simulink model "mcb_ipmsm_pos_est_f28379d"  (R2023b)
settings: Solver=FixedStepDiscrete  StartTime=0.0  StopTime=1  RelTol=1e-3  EnableMultiTasking=on
InitFcn:
  | mcb_ipmsm_pos_est_f28379d_data;
  | init_ang = eval(get_param([bdroot '/Inverter and Motor/Simulation/Init angle'],'Value'))/pmsm.p;
values from neighbouring files (symbols this model uses):
  dataType = 'single'    [mcb_ipmsm_pos_est_f28379d_data.m]
  inverter = mcb_updateInverterParameters(pmsm,inverter,target)    [mcb_ipmsm_pos_est_f28379d_data.m]
  pmsm = mcb_SetPMSMMotorParameters('Teknic2310P')    [mcb_ipmsm_pos_est_f28379d_data.m]
  PWM_frequency = 20e3    (= 20000)    [mcb_ipmsm_pos_est_f28379d_data.m]
  target = mcb_SetProcessorDetails('F28379D',PWM_frequency)    [mcb_ipmsm_pos_est_f28379d_data.m]
  Ts = T_pwm    (= 5e-05)    [mcb_ipmsm_pos_est_f28379d_data.m]
  Ts_motor_simscape = T_pwm/2000    (= 2.5e-08)    [mcb_ipmsm_pos_est_f28379d_data.m]
  Ts_simulink = T_pwm/2    (= 2.5e-05)    [mcb_ipmsm_pos_est_f28379d_data.m]
undefined symbols (not defined in the file or in its folder): Down, GPTRIP1SEL, GPTRIP2SEL, PU_System, TZ1, TZ2, Up
libraries: nesl_utility x12, c2802xlib x7, fl_lib x7, c280xlib x5, ee_lib x5, c2837xDlib x4, simulink x3, svdschedulerlib x1, mcbcontrolslib x1, mcbsensorlessestimatorlib x1, svdutilitieslib x1, mcbpositiondecoderlib x1
(part 1 of 2)
settings Model: ExtModeTrigDuration=8  Creator=The MathWorks, Inc.  LastModifiedBy=The MathWorks, Inc.
settings SolverCC: AlgebraicLoopSolver=TrustRegion  MaxZcPerStep=1
settings DataIOCC: ReturnWorkspaceOutputs=off
settings OptimizationCC: DefaultParameterBehavior=Inlined  DefaultUnderspecifiedDataType=single  OptimizeBlockIOStorage=off  ReuseModelBlockBuffer=off  EnhancedBackFolding=on  InitFltsAndDblsToZero=on  NoFixptDivByZeroProtection=on  EfficientFloat2IntCast=on  EfficientMapNaN2IntZero=off  MaxStackSize=1024  OptimizeBlockOrder=speed  DifferentSizesBufferReuse=on  DenormalBehavior=FlushToZero  EfficientTunableParamExpr=on
settings DebuggingCC: ReadBeforeWriteMsg=DisableAll  WriteAfterWriteMsg=DisableAll  WriteAfterReadMsg=DisableAll  InheritedTsInSrcMsg=none  MultiTaskDSMMsg=none  ParameterPrecisionLossMsg=none  ParameterTunabilityLossMsg=error  UnconnectedInputMsg=warning  UnconnectedOutputMsg=warning  UnconnectedLineMsg=warning
settings HardwareCC: ProdBitPerChar=16  ProdBitPerInt=16  ProdBitPerPointer=32  ProdBitPerSizeT=32  ProdBitPerPtrDiffT=32  ProdLargestAtomicInteger=Integer  ProdLargestAtomicFloat=None  ProdWordSize=16  ProdLongLongMode=on  ProdHWDeviceType=Texas Instruments->C2000
settings ModelReferenceCC: EnableRefExpFcnMdlSchedulingChecks=on
settings SFSimCC: MATLABDynamicMemAlloc=off
settings RTWCC: Description=Embedded Coder  SystemTargetFile=ert.tlc  HardwareBoard=TI Delfino F28379D LaunchPad  TemplateMakefile=ert_default_tmf  GenerateReport=on  Toolchain=Texas Instruments Code Composer Studio (C2000)  DLArmComputeVersion=19.05
settings CodeAppCC: IgnoreCustomStorageClasses=off  StateflowObjectComments=on
settings ERTTargetCC: CodeReplacementLibrary=TI C28x  ExtModeStaticAllocSize=10000  ConvertIfToSwitch=off  SuppressUnreachableDefaultCases=off  MemSecPackage=tic2000demospkg

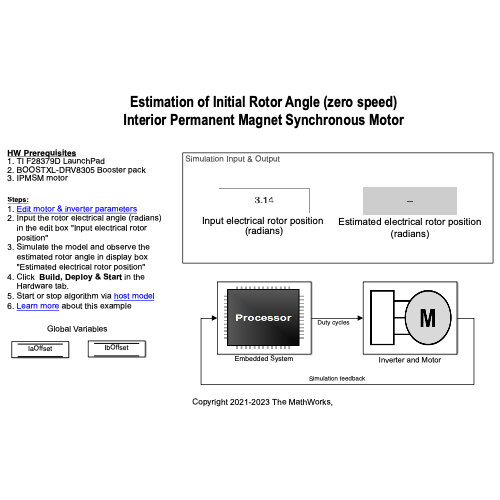
[thumbnail: Simulink's stored preview of the top-level diagram]
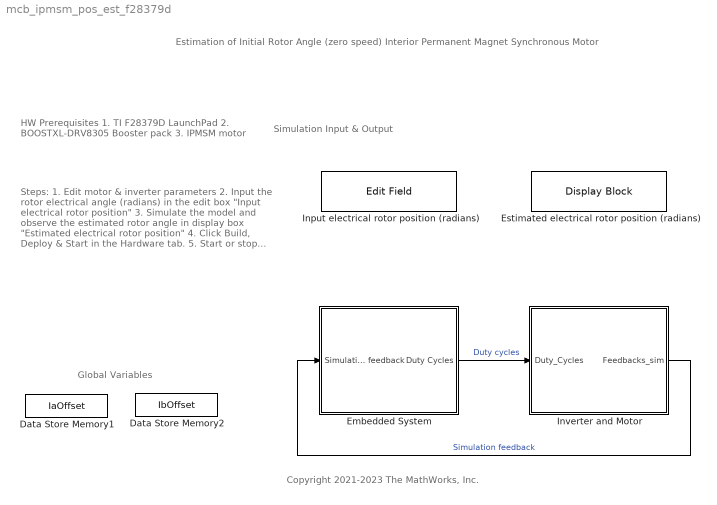
== system mcb_ipmsm_pos_est_f28379d ==
  note: Estimation of Initial Rotor Angle (zero speed)
      | Interior Permanent Magnet Synchronous Motor
  note: Simulation Input & Output
  note: Steps:
      | 1. Edit motor & inverter parameters
      | 2. Input the rotor electrical angle (radians)
      | in the edit box "Input electrical rotor
      | position"
      | 3. Simulate the model and observe the
      | estimated rotor angle in display box
      | "Estimated electrical rotor position"
      | 4. Click Build, Deploy & Start in the
      | Hardware tab.
      | 5. Start or stop algorithm via host model
      | 6. Learn more about this example
  note: HW Prerequisites
      | 1. TI F28379D LaunchPad
      | 2. BOOSTXL-DRV8305 Booster pack
      | 3. IPMSM motor
  note: Global Variables
  note: Copyright 2021-2023 The MathWorks, Inc.
  Data Store Memory1 : DataStoreMemory  DataStoreName=IaOffset  InitialValue=inverter.CtSensAOffset  ShowAdditionalParam=off
  Data Store Memory2 : DataStoreMemory  DataStoreName=IbOffset  InitialValue=inverter.CtSensBOffset  ShowAdditionalParam=off
  Embedded System : Subsystem
      mask Display: image('mcb_pmsmfoc_processor.png'); % Use "Edit Image" on toolstrip to change.
  Estimated electrical rotor position (radians) : DisplayBlock  LabelPosition=Hide  Transparency=1  FormatString=%5d
  Input electrical rotor position (radians) : EditField  LabelPosition=Hide  ShowInitialText=on  Alignment=Center
  Inverter and Motor : Subsystem
      mask Display: image('mcb_pmsmfoc_motor.png'); % Use "Edit Image" on toolstrip to change.
  wires:
  Inverter and Motor/1(Feedbacks_sim) -> Embedded System/1(Simulation feedback)  "Simulation feedback"
  Embedded System/1(Duty Cycles) -> Inverter and Motor/1(Duty_Cycles)  "Duty cycles"

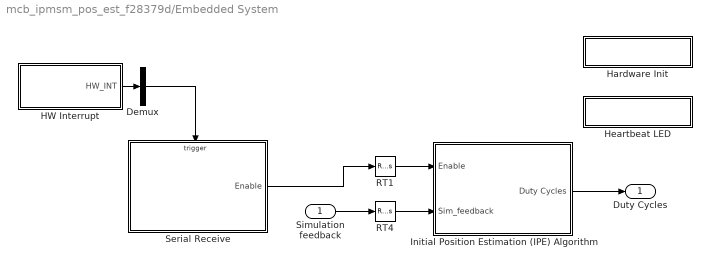
== system mcb_ipmsm_pos_est_f28379d/Embedded System ==
  Simulation feedback : Inport
  Demux : Demux  Outputs=1
  HW Interrupt : Subsystem  Variant=on  VariantControlMode=sim codegen switching
  Hardware Init : Subsystem  TreatAsAtomicUnit=on
  Heartbeat LED : Subsystem  TreatAsAtomicUnit=on
  Initial Position Estimation (IPE) Algorithm : Subsystem
      settings: RTWSystemCode=Nonreusable function
  RT1 : RateTransition  Deterministic=off  OutPortSampleTime=Ts
  RT4 : RateTransition  Deterministic=off  OutPortSampleTime=Ts
  Serial Receive : Subsystem  SystemSampleTime=1e-3
  Duty Cycles : Outport
  wires:
  HW Interrupt/1(HW_INT) -> Demux/1
  RT4/1 -> Initial Position Estimation (IPE) Algorithm/2(Sim_feedback)
  Initial Position Estimation (IPE) Algorithm/1(Duty Cycles) -> Duty Cycles/1
  Simulation feedback/1 -> RT4/1
  Demux/1 -> Serial Receive/Trigger
  Serial Receive/1(Enable) -> RT1/1
  RT1/1 -> Initial Position Estimation (IPE) Algorithm/1(Enable)

== system mcb_ipmsm_pos_est_f28379d/Inverter and Motor ==
  Duty_Cycles : Inport
  Codegeneration : Subsystem
  Simulation : Subsystem
  Variant Sink : VariantSink  VariantControlMode=sim codegen switching
  Variant Source : VariantSource  VariantControlMode=sim codegen switching
  Feedbacks_sim : Outport  VectorParamsAs1DForOutWhenUnconnected=off
  wires:
  Duty_Cycles/1 -> Variant Sink/1
  Variant Source/1 -> Feedbacks_sim/1
  Variant Sink/2 -> Simulation/1(Duty_Cycles)
  Simulation/1(Feedbacks) -> Variant Source/2
  Variant Sink/1 -> Codegeneration/1(Duty_Cycles)
  Codegeneration/1(Feedbacks) -> Variant Source/1

== system mcb_ipmsm_pos_est_f28379d/Embedded System/HW Interrupt ==
  Code generation : Subsystem  VariantControl=(codegen)
  Simulation : Subsystem  VariantControl=(sim)
  HW_INT : Outport  OutputFunctionCall=on

== system mcb_ipmsm_pos_est_f28379d/Embedded System/Hardware Init ==
  6PWM_Mode : Constant  Priority=1000  Value=0x3A16  OutDataTypeStr=uint16  SampleTime=-1
  ADC_Gain_Setting : Constant  Priority=1000  Value=inverter.SPI_Gain_Setting  OutDataTypeStr=uint16  SampleTime=-1
  Event Listener : EventListener  DisableCoverage=on  EventName=reset
  Mux : Mux  Inputs=2
  Variant Subsystem : Subsystem  Variant=on  VariantControlMode=sim codegen switching
  wires:
  6PWM_Mode/1 -> Mux/1
  ADC_Gain_Setting/1 -> Mux/2
  Mux/1 -> Variant Subsystem/1(In1)

== system mcb_ipmsm_pos_est_f28379d/Embedded System/Heartbeat LED ==
  note: Heartbeat LED 1HZ
  Heartbeat LED : Subsystem  Variant=on  VariantControlMode=sim codegen switching
  RED_LED : Constant  OutDataTypeStr=uint16  SampleTime=0.5
  wires:
  RED_LED/1 -> Heartbeat LED/1(In1)

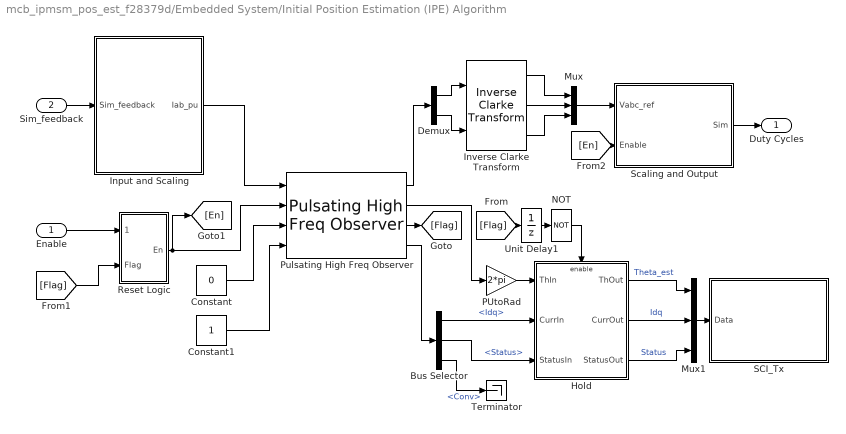
== system mcb_ipmsm_pos_est_f28379d/Embedded System/Initial Position Estimation (IPE) Algorithm ==
  Enable : Inport
  Sim_feedback : Inport  Port=2
  Bus Selector : BusSelector  OutputSignals=Idq,Status,Conv
  Constant : Constant  Value=0  OutDataTypeStr=dataType
  Constant1 : Constant  OutDataTypeStr=boolean
  Demux : Demux  Outputs=2
  Hold : Subsystem
  Input and Scaling : Subsystem
  Inverse Clarke Transform : mcbcontrolslib/Inverse Clarke Transform  PhaseInput=Two inputs  EnPowerInv=off
  Mux : Mux  Inputs=3
  Mux1 : Mux  Inputs=3
  NOT : Logic  Operator=NOT  IconShape=distinctive  AllPortsSameDT=off  OutDataTypeStr=boolean
  PUtoRad : Gain  Gain=2*pi  OutDataTypeStr=Inherit: Same as input
  Pulsating High Freq Observer : mcbsensorlessestimatorlib/Pulsating High Freq Observer  BlkSampleTime=Ts  InputUnit=Per-unit  dataType=dataType  AutoDefaultPHF=off  AutoDefaultDP=off  StatorResistance=pmsm.Rs  StatorDaxisInductance=pmsm.Ld  StatorQaxisInductance=pmsm.Lq  BaseVoltage=PU_System.V_base  BaseCurrent=PU_System.I_base  Voltphf=0.5  Frqphf=2000  Cfrqphf=131.9037  SelectForTuning=Controller gains  Kp=1954.6647  Ki=7392.5303  Tsettling=0.66794  DampingRatio=0.99  Tophf=0.0066794  Tcphf=0.66794  Idlephf=0.0066794  Threshold=4e-4  Voltdp=0.5  Tdp=0.00066955  Idledp=50e-3  PHF_OpenLoop=134  PHF_Period=10  PHF_Delay=134  PHF_OL_Total=804  PHF_CloseLoop=13359  PHF_Total=14297  DP_On=14  DP_Delay=1000  DP_Total=0  IPE_Total=16325  DefaultCal=0
      settings: RTWMemSecFuncExecute=code_ramfuncs
  Reset Logic : Subsystem
  SCI_Tx : Subsystem  Variant=on  VariantControlMode=sim codegen switching
  Scaling and Output : Subsystem
  Terminator : Terminator
  Unit Delay1 : UnitDelay  SampleTime=-1  HasFrameUpgradeWarning=on
  Duty Cycles : Outport  InitialOutput=0  VectorParamsAs1DForOutWhenUnconnected=off
  wires:
  Mux1/1 -> SCI_Tx/1(Data)
  Sim_feedback/1 -> Input and Scaling/1(Sim_feedback)
  Scaling and Output/1(Sim) -> Duty Cycles/1
  Inverse Clarke Transform/1 -> Mux/1
  Inverse Clarke Transform/2 -> Mux/2
  Inverse Clarke Transform/3 -> Mux/3
  Mux/1 -> Scaling and Output/1(Vabc_ref)
  Demux/1 -> Inverse Clarke Transform/1
  Demux/2 -> Inverse Clarke Transform/2
  Pulsating High Freq Observer/1 -> Demux/1
  [En] -> Scaling and Output/2(Enable)
  Input and Scaling/1(Iab_pu) -> Pulsating High Freq Observer/1
  Pulsating High Freq Observer/2 -> PUtoRad/1
  Hold/1(ThOut) -> Mux1/1  "Theta_est"
  NOT/1 -> Hold/Enable
  Constant/1 -> Pulsating High Freq Observer/3
  Constant1/1 -> Pulsating High Freq Observer/4
  Pulsating High Freq Observer/4 -> Bus Selector/1
  Pulsating High Freq Observer/3 -> [Flag]
  Enable/1 -> Reset Logic/1(Enable)
  [Flag] -> Reset Logic/2(Flag)
  Reset Logic/1(En) -> Pulsating High Freq Observer/2, [En]
  Bus Selector/1 -> Hold/2(CurrIn)  "<Idq>"
  Bus Selector/2 -> Hold/3(StatusIn)  "<Status>"
  Hold/3(StatusOut) -> Mux1/3  "Status"
  [Flag] -> Unit Delay1/1
  Unit Delay1/1 -> NOT/1
  Hold/2(CurrOut) -> Mux1/2  "Idq"
  Bus Selector/3 -> Terminator/1  "<Conv>"
  PUtoRad/1 -> Hold/1(ThIn)

== system mcb_ipmsm_pos_est_f28379d/Embedded System/Serial Receive ==
  SCI_Rx_INT : TriggerPort  TriggerType=function-call  VariantControl=Variant
  Data Type Conversion1 : DataTypeConversion  OutDataTypeStr=boolean  RndMeth=Simplest  SaturateOnIntegerOverflow=off
  Data_Conditioning_Rx : Subsystem  Variant=on
  SCi_Rx : Subsystem  Variant=on  VariantControlMode=sim codegen switching
  Enable : Outport
  wires:
  SCi_Rx/1(Data) -> Data_Conditioning_Rx/1(In1)
  Data_Conditioning_Rx/1(Out3) -> Data Type Conversion1/1
  Data Type Conversion1/1 -> Enable/1

== system mcb_ipmsm_pos_est_f28379d/Inverter and Motor/Codegeneration ==
  Duty_Cycles : Inport
  Ground : Ground
  Terminator : Terminator
  Feedbacks : Outport  VectorParamsAs1DForOutWhenUnconnected=off
  wires:
  Duty_Cycles/1 -> Terminator/1
  Ground/1 -> Feedbacks/1

== system mcb_ipmsm_pos_est_f28379d/Inverter and Motor/Simulation ==
  note: "Initi angle" constant is connected with user input " Input electrical rotor
      | position " to define initial rotor position for PMSM motor block
  Duty_Cycles : Inport
  Constant : Constant  Value=0  OutDataTypeStr=dataType
  Data Type Conversion : DataTypeConversion  OutDataTypeStr=single  RndMeth=Simplest  SaturateOnIntegerOverflow=off
  Init angle : Constant  Value=3.14  OutDataTypeStr=dataType
  Inveter and Motor : Subsystem  VariantControl=(get_param([bdroot '/MotorWindingType'], 'Value') == '1')
  RT1 : RateTransition  Deterministic=off  OutPortSampleTime=Ts_simulink
  Sensor_Measurements : Subsystem
  Terminator2 : Terminator
  Feedbacks : Outport  VectorParamsAs1DForOutWhenUnconnected=off
  wires:
  Sensor_Measurements/1(Sim_fb) -> Feedbacks/1
  RT1/1 -> Sensor_Measurements/1(PhaseCurr)
  Duty_Cycles/1 -> Data Type Conversion/1
  Constant/1 -> Inveter and Motor/2(Load)
  Inveter and Motor/1(Iabc) -> RT1/1
  Init angle/1 -> Terminator2/1
  Data Type Conversion/1 -> Inveter and Motor/1(Vabc_In_PU)

== system mcb_ipmsm_pos_est_f28379d/Embedded System/HW Interrupt/Code generation ==
  HWI_SCIA_RX_INT : svdschedulerlib/Hardware Interrupt v2  ISRGroup=ADC - Analog to Digital Converter  ISRName=ADCA1_INT  ISRNumber=32  NumEventsToServe=1  EventsList={'on','EOC event','1';'off','Overflow event','2';'off','Custom event','3'}  SelectedEvents={'event1'}  TaskPriority=50  DisablePreemption=on  ClearInterruptFlagsAtEndOfEvent=on  InterruptDefinitionFile=$(TARGET_ROOT)/registry/interrupts/F2837xS_interrupts.xml  HardwareBoard=F2837x  EnableSimPort=off
      settings: LibrarySourceBlock=c2000lib/Scheduling/Hardware Interrupt
  HW_INT : Outport
  wires:
  HWI_SCIA_RX_INT/1 -> HW_INT/1

== system mcb_ipmsm_pos_est_f28379d/Embedded System/HW Interrupt/Simulation ==
  SCI_Rx_INT : simulink/Ports & Subsystems/Function-Call Generator  sample_time=0.1  numberOfIterations=1  DisallowWideOutput=off
  HW_INT : Outport
  wires:
  SCI_Rx_INT/1 -> HW_INT/1

== system mcb_ipmsm_pos_est_f28379d/Embedded System/Hardware Init/Variant Subsystem ==
  In1 : Inport
  Code Generation : Subsystem  VariantControl=(codegen)
  Simulation : Subsystem  VariantControl=(sim)

== system mcb_ipmsm_pos_est_f28379d/Embedded System/Heartbeat LED/Heartbeat LED ==
  In1 : Inport
  Code generation : Subsystem  VariantControl=(codegen)
  Simulation : Subsystem  VariantControl=(sim)

== system mcb_ipmsm_pos_est_f28379d/Embedded System/Initial Position Estimation (IPE) Algorithm/Hold ==
  ThIn : Inport
  CurrIn : Inport  Port=2
  StatusIn : Inport  Port=3
  Enable : EnablePort
  ThOut : Outport
  CurrOut : Outport  Port=2
  StatusOut : Outport  Port=3
  wires:
  ThIn/1 -> ThOut/1
  CurrIn/1 -> CurrOut/1
  StatusIn/1 -> StatusOut/1

== system mcb_ipmsm_pos_est_f28379d/Embedded System/Initial Position Estimation (IPE) Algorithm/Input and Scaling ==
  note: HW Driver Blocks
  Sim_feedback : Inport
  Demux1 : Demux  Outputs=2
  HW_Inputs : Subsystem  Variant=on  VariantControlMode=sim codegen switching
  Input Scaling : Subsystem
  Iab_pu : Outport
  wires:
  Demux1/2 -> Input Scaling/2(Ib_ADC)
  Demux1/1 -> Input Scaling/1(Ia_ADC)
  HW_Inputs/1(Out) -> Demux1/1
  Sim_feedback/1 -> HW_Inputs/1(Sim)
  Input Scaling/1(Iab_pu) -> Iab_pu/1

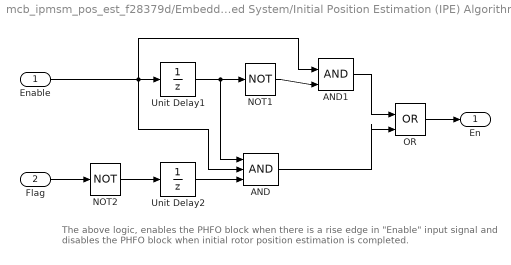
== system mcb_ipmsm_pos_est_f28379d/Embedded System/Initial Position Estimation (IPE) Algorithm/Reset Logic ==
  note: The above logic, enables the PHFO block when there is a rise edge in "Enable" input signal and disables the PHFO block when initial rotor position estimation is completed.
  Enable : Inport
  Flag : Inport  Port=2
  AND : Logic  Inputs=3  IconShape=distinctive  AllPortsSameDT=off  OutDataTypeStr=boolean
  AND1 : Logic  IconShape=distinctive  AllPortsSameDT=off  OutDataTypeStr=boolean
  NOT1 : Logic  Operator=NOT  IconShape=distinctive  AllPortsSameDT=off  OutDataTypeStr=boolean
  NOT2 : Logic  Operator=NOT  IconShape=distinctive  AllPortsSameDT=off  OutDataTypeStr=boolean
  OR : Logic  Operator=OR  IconShape=distinctive  AllPortsSameDT=off  OutDataTypeStr=boolean
  Unit Delay1 : UnitDelay  SampleTime=-1  HasFrameUpgradeWarning=on
  Unit Delay2 : UnitDelay  SampleTime=-1  HasFrameUpgradeWarning=on
  En : Outport
  wires:
  Flag/1 -> NOT2/1
  AND/1 -> OR/2
  AND1/1 -> OR/1
  Enable/1 -> AND/2, AND1/1, Unit Delay1/1
  NOT1/1 -> AND1/2
  OR/1 -> En/1
  NOT2/1 -> Unit Delay2/1
  Unit Delay2/1 -> AND/3
  Unit Delay1/1 -> NOT1/1, AND/1

== system mcb_ipmsm_pos_est_f28379d/Embedded System/Initial Position Estimation (IPE) Algorithm/SCI_Tx ==
  Data : Inport
  Code Generation : Subsystem  VariantControl=(codegen)
  Simulation : Subsystem  VariantControl=(sim)

== system mcb_ipmsm_pos_est_f28379d/Embedded System/Initial Position Estimation (IPE) Algorithm/Scaling and Output ==
  note: HW Driver Blocks
  Vabc_ref : Inport
  Enable : Inport  Port=2
  HW_Outputs : Subsystem  Variant=on  VariantControlMode=sim codegen switching
  Mux : Mux  Inputs=2
  Output Scaling : Subsystem
  Sim : Outport
  wires:
  Mux/1 -> HW_Outputs/1(Inverter Signals)
  Output Scaling/2(PWM_Enable) -> Mux/2
  Output Scaling/1(PWM_Duty_Cycles) -> Mux/1
  Vabc_ref/1 -> Output Scaling/1(Vabc_ref)
  HW_Outputs/1(Sim) -> Sim/1
  Enable/1 -> Output Scaling/2(Enable)

== system mcb_ipmsm_pos_est_f28379d/Embedded System/Serial Receive/Data_Conditioning_Rx ==
  In1 : Inport
  Data_Type_Fixed_Point : Subsystem  VariantControl=~isequal(dataType, 'single')
  Data_Type_Float : Subsystem  VariantControl=isequal(dataType, 'single')
  Out3 : Outport

== system mcb_ipmsm_pos_est_f28379d/Embedded System/Serial Receive/SCi_Rx ==
  Code Generation : Subsystem  Variant=on  VariantControl=(codegen)
  Simulation : Subsystem  VariantControl=(sim)
  Data : Outport

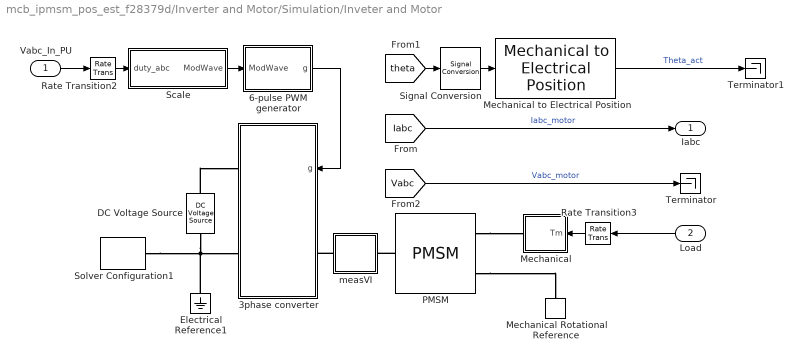
== system mcb_ipmsm_pos_est_f28379d/Inverter and Motor/Simulation/Inveter and Motor ==
  Vabc_In_PU : Inport
  Load : Inport  Port=2
  3phase converter : Subsystem
  6-pulse PWM generator : Subsystem  mask{fs=PWM_frequency}
      mask prompts: fs "Carrier Frequency (Hz)"
  DC Voltage Source : fl_lib/Electrical/Electrical Sources/DC Voltage Source  v0=inverter.V_dc V
  Electrical Reference1 : fl_lib/Electrical/Electrical Elements/Electrical Reference
  Mechanical : Subsystem
  Mechanical Rotational Reference : fl_lib/Mechanical/Rotational Elements/Mechanical Rotational Reference
  Mechanical to Electrical Position : mcbpositiondecoderlib/Mechanical to Electrical Position  PolePairsInputType=Specify via dialog  NrPP=pmsm.p  selectedRange=Radians  MechOfstInputType=Specify via dialog  mechOffsetIn=0  maxAngleIn=2*pi  InputDataType=dataType  VariantSelect=floating-point
  PMSM : ee_lib/Electromechanical/Permanent Magnet/PMSM  port_option=ee.enum.threePhasePort.composite  winding_type=ee.enum.statorconnection.delta  machine_param=ee.enum.pmsm.parameterization.tabulated  nPolePairs=pmsm.p  pmflux_param=ee.enum.pmflux.fluxlinkage  pm_flux_linkage=pmsm.FluxPM Wb  torque_constant=0.18 N*m/A  back_emf_constant=0.18 V/(rad/s)  stator_param=ee.enum.statorparam.LdLqL0  Ld=pmsm.Ld H  Lq=pmsm.Lq H  idVec=pmsm.nonlin.idVec A  iqVec=pmsm.nonlin.iqVec A  LdMatrix=pmsm.nonlin.LdMatrix H  LqMatrix=pmsm.nonlin.LqMatrix H  PmMatrix=pmsm.nonlin.PmMatrix Wb  ktMatrix=0.18 * ones(3, 3) N*m/A  keMatrix=0.18 * ones(3, 3) V/(rad/s)  L0=0 H  Ls=0.0002 H  Lm=-0.00002 H  Ms=0.00002 H  Rs=pmsm.PhaseResFactor*pmsm.Rs Ohm  zero_sequence=ee.enum.park.zerosequence.exclude  axes_param=ee.enum.rotorangle.daxis  loss_param=ee.enum.ironloss.none  losses_oc=[0, 0, 0] W  losses_sc=[0, 0, 0] W  f_losses=60 Hz  Isc_losses=95 A  J=pmsm.J kg*m^2  lam=pmsm.B N*m/(rad/s)  i_d_specify=off  i_d_priority=None  i_d=0 A  i_d_nominal_specify=off  i_d_nominal_unit=A  i_d_nominal_value=1  i_q_specify=off  i_q_priority=None  i_q=0 A  i_q_nominal_specify=off  i_q_nominal_unit=A  i_q_nominal_value=1  torque_specify=off  torque_priority=None  torque=0 N*m  torque_nominal_specify=off  torque_nominal_unit=N*m  torque_nominal_value=1  angular_velocity_specify=off  angular_velocity_priority=High  angular_velocity=0 rpm  angular_velocity_nominal_specify=off  angular_velocity_nominal_unit=rpm  angular_velocity_nominal_value=1  angular_position_specify=on  angular_position_priority=High  angular_position=init_ang+pmsm.PositionOffset rad  angular_position_nominal_specify=off  angular_position_nominal_unit=deg  angular_position_nominal_value=1  alpha=3.93e-3 1/K  alpha_flux=-0.001 1/K  Tmeas=298.15 K  stator_thermal_mass=100 J/K  rotor_thermal_mass=200 J/K  Rm_percent_rotor=90  Rd_percent_rotor=30  temperatureA_specify=off  temperatureA_priority=High  temperatureA=25 degC  temperatureA_nominal_specify=off  temperatureA_nominal_unit=degC  temperatureA_nominal_value=1  temperatureB_specify=off  temperatureB_priority=High  temperatureB=25 degC  temperatureB_nominal_specify=off  temperatureB_nominal_unit=degC  temperatureB_nominal_value=1  temperatureC_specify=off  temperatureC_priority=High  temperatureC=25 degC  temperatureC_nominal_specify=off  temperatureC_nominal_unit=degC  temperatureC_nominal_value=1  temperatureR_specify=off  temperatureR_priority=High  temperatureR=25 degC  temperatureR_nominal_specify=off  temperatureR_nominal_unit=degC  temperatureR_nominal_value=1
      settings: InternalSimscapePortConfiguration="{\"Bottom\":[],\"Left\":[{\"id\":\"N\",\"label\":\"~\",\"type\":\"foundation.electrical.three_phase\"}],\"Right\":[{\"id\":\"R\",\"label\":\"R\",\"type\":\"foundation.mechanical.rotational.rotational\"},{\"id\":\"C\",\"label\":\"C\",\"type\":\"foundation.mechanical.rotational.rotational\"}],\"Top\":[]}"
  Rate Transition2 : RateTransition  Deterministic=off  OutPortSampleTime=Ts_motor_simscape
  Rate Transition3 : RateTransition  Deterministic=off  OutPortSampleTime=Ts_motor_simscape
  Scale : Subsystem
  Signal Conversion : SignalConversion  OverrideOpt=off
  Solver Configuration1 : nesl_utility/Solver Configuration  PhysicalDomain=network_engine_domain  SubClassName=solver  LeftPortType=input  RightPortType=generic  Tones=[]  Harmonics=[]  SimulateNoise=off  Profile=off  UseLocalSampling=off  EnableSwitchedLinearOptims=on  FrequencyDomain=off  UseCCode=off  RelTol=0.001  AbsTol=0.001  MinStep=1e-09  ToWorkspace=off  RevertToSquareIcSolve=off  NumHomotopyIterations=100  PhasorMode=off  PhasorModeNumHarmonics=1  ConsistencySolver=NEWTON_XTOL_AFTER_FTOL  IndexReductionMethod=DerivativeReplacement  DoDC=off  ResidualTolerance=1e-09  ConsistencyTolSource=GLOBAL  ConsistencyAbsTol=0.001  ConsistencyRelTol=0.001  ConsistencyTolFactor=1e-09  UseLocalSolver=on  LocalSolverChoice=NE_PARTITIONING_ADVANCER  ResolveIndetEquations=on  FunctionEvalNumThread=1  LocalSolverSampleTime=Ts_motor_simscape  DoFixedCost=on  MaxNonlinIter=3  MaxModeIter=2  ComputeImpulses=off  ImpulseIterations=2  LinearAlgebra=Sparse  LinearAlgebraNumThread=0  EquationFormulation=NE_TIME_EF  DelaysMemoryBudget=1024  AutomaticFiltering=off  FilteringTimeConstant=0.001  PartitionStorageMethod=AS_NEEDED  PartitionMemoryBudget=1024  PartitionMethod=ROBUST  MultibodyUseLocalSolver=off  MultibodyLocalSolverChoice=ODE1  MultibodyLocalSolverSampleTime=0.001
  Terminator : Terminator
  Terminator1 : Terminator
  measVI : Subsystem
  Iabc : Outport
  wires:
  Load/1 -> Rate Transition3/1
  6-pulse PWM generator/1(g) -> 3phase converter/1(g)
  Scale/1(ModWave) -> 6-pulse PWM generator/1(ModWave)
  Rate Transition2/1 -> Scale/1(duty_abc)
  Rate Transition3/1 -> Mechanical/1(Tm)
  [Vabc] -> Terminator/1  "Vabc_motor"
  [Iabc] -> Iabc/1  "Iabc_motor"
  Vabc_In_PU/1 -> Rate Transition2/1
  Signal Conversion/1 -> Mechanical to Electrical Position/1
  [theta] -> Signal Conversion/1
  Mechanical to Electrical Position/1 -> Terminator1/1  "Theta_act"
  connections:
  DC Voltage Source/RConn1 -- Solver Configuration1/RConn1 -- Electrical Reference1/LConn1 -- 3phase converter/RConn2
  measVI/LConn1 -- 3phase converter/LConn1
  DC Voltage Source/LConn1 -- 3phase converter/RConn1
  PMSM/LConn1 -- measVI/RConn1
  PMSM/RConn1 -- Mechanical/RConn1
  PMSM/RConn2 -- Mechanical Rotational Reference/LConn1

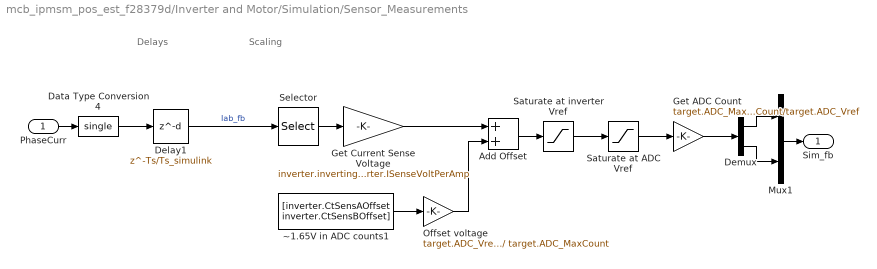
== system mcb_ipmsm_pos_est_f28379d/Inverter and Motor/Simulation/Sensor_Measurements ==
  note: Scaling
  note: Delays
  PhaseCurr : Inport
  Add Offset : Sum  RndMeth=Simplest
  Data Type Conversion4 : DataTypeConversion  OutDataTypeStr=single  RndMeth=Simplest  SaturateOnIntegerOverflow=off
  Delay1 : Delay  DelayLength=Ts/Ts_simulink
  Demux : Demux  Outputs=2
  Get ADC Count : Gain  Gain=target.ADC_MaxCount/target.ADC_Vref  OutMin=0  OutMax=target.ADC_MaxCount  OutDataTypeStr=uint16  RndMeth=Simplest
  Get Current Sense Voltage : Gain  Gain=inverter.invertingAmp * inverter.ISenseVoltPerAmp  RndMeth=Simplest  OutDataTypeStr=Inherit: Same as input
  Mux1 : Mux  Inputs=2
  Offset voltage : Gain  Gain=target.ADC_Vref / target.ADC_MaxCount  RndMeth=Simplest
  Saturate at ADC Vref : Saturate  UpperLimit=target.ADC_Vref  LowerLimit=0
  Saturate at inverter Vref : Saturate  UpperLimit=inverter.ISenseVref  LowerLimit=0
  Selector : Selector  InputPortWidth=3  IndexOptions=Index vector (dialog)  Indices=[1 2]  OutputSizes=1
  ~1.65V in ADC counts1 : Constant  Value=[inverter.CtSensAOffset inverter.CtSensBOffset]  OutDataTypeStr=single  SampleTime=-1
  Sim_fb : Outport  VectorParamsAs1DForOutWhenUnconnected=off
  wires:
  Delay1/1 -> Selector/1  "Iab_fb"
  Data Type Conversion4/1 -> Delay1/1
  PhaseCurr/1 -> Data Type Conversion4/1
  Demux/1 -> Mux1/1
  Mux1/1 -> Sim_fb/1
  Demux/2 -> Mux1/2
  ~1.65V in ADC counts1/1 -> Offset voltage/1
  Get Current Sense Voltage/1 -> Add Offset/1
  Saturate at ADC Vref/1 -> Get ADC Count/1
  Saturate at inverter Vref/1 -> Saturate at ADC Vref/1
  Offset voltage/1 -> Add Offset/2
  Add Offset/1 -> Saturate at inverter Vref/1
  Get ADC Count/1 -> Demux/1
  Selector/1 -> Get Current Sense Voltage/1

== system mcb_ipmsm_pos_est_f28379d/Embedded System/Hardware Init/Variant Subsystem/Code Generation ==
  note: for BoostXL-DRV8305 connected to LaunchXL-28379D
  note: System Outputs
  note: Enable ADC offset calibration only when motor is not loaded and not rotating due to external factors
  In1 : Inport
  ADC Calib Enable : Constant  Value=inverter.ADCOffsetCalibEnable  OutDataTypeStr=Inherit: Inherit via back propagation
  "Calculate ADC Offset " : Subsystem  Priority=1001  TreatAsAtomicUnit=on
  DRV Enable : Subsystem  Priority=1
  Default ADC Offset : Subsystem  Priority=1001  TreatAsAtomicUnit=on
  NOT : Logic  Operator=NOT  IconShape=distinctive  AllPortsSameDT=off  OutDataTypeStr=boolean
  wires:
  In1/1 -> DRV Enable/1(In)
  NOT/1 -> Default ADC Offset/Enable
  ADC Calib Enable/1 -> NOT/1, "Calculate ADC Offset "/Enable

== system mcb_ipmsm_pos_est_f28379d/Embedded System/Hardware Init/Variant Subsystem/Simulation ==
  In1 : Inport
  Terminator : Terminator
  wires:
  In1/1 -> Terminator/1

== system mcb_ipmsm_pos_est_f28379d/Embedded System/Heartbeat LED/Heartbeat LED/Code generation ==
  In1 : Inport
  Digital Output : c2837xDlib/Digital Output  GPIO_Number=GPIO32~GPIO39  GPIO_Bit0=off  GPIO_BIT0_Toggle=on  GPIO_Bit1=off  GPIO_BIT1_Toggle=off  GPIO_Bit2=on  GPIO_BIT2_Toggle=on  GPIO_Bit3=off  GPIO_BIT3_Toggle=off  GPIO_Bit4=off  GPIO_BIT4_Toggle=off  GPIO_Bit5=off  GPIO_BIT5_Toggle=off  GPIO_Bit6=off  GPIO_BIT6_Toggle=off  GPIO_Bit7=off  GPIO_BIT7_Toggle=off
  wires:
  In1/1 -> Digital Output/1

== system mcb_ipmsm_pos_est_f28379d/Embedded System/Heartbeat LED/Heartbeat LED/Simulation ==
  In1 : Inport
  Simulation_Terminator : Terminator
  wires:
  In1/1 -> Simulation_Terminator/1

== system mcb_ipmsm_pos_est_f28379d/Embedded System/Initial Position Estimation (IPE) Algorithm/Input and Scaling/HW_Inputs ==
  Sim : Inport
  Sensor Driver Blocks (codegen) : Subsystem  VariantControl=(codegen)
  Sensor Driver Blocks (sim) : Subsystem  VariantControl=(sim)
  Out : Outport

== system mcb_ipmsm_pos_est_f28379d/Embedded System/Initial Position Estimation (IPE) Algorithm/Input and Scaling/Input Scaling ==
  note: Current Measurements
  Ia_ADC : Inport
  Ib_ADC : Inport  Port=2
  Calculate Phase Currents : Subsystem
  Iab_pu : Outport
  wires:
  Ia_ADC/1 -> Calculate Phase Currents/1(Ia_ADC)
  Ib_ADC/1 -> Calculate Phase Currents/2(Ib_ADC)
  Calculate Phase Currents/1(Iab_pu) -> Iab_pu/1

== system mcb_ipmsm_pos_est_f28379d/Embedded System/Initial Position Estimation (IPE) Algorithm/SCI_Tx/Code Generation ==
  Data : Inport
  Data_Conditioning_Tx : Subsystem  Variant=on
  Data_Logging : Subsystem
  Demux2 : Demux  Outputs=2
  While Iterator Subsystem : Subsystem  TreatAsAtomicUnit=on
  wires:
  Data_Conditioning_Tx/1(Data_Log) -> Data_Logging/1(Data_Log)
  Demux2/1 -> While Iterator Subsystem/1(Data)  "SCI_Tx_Data"
  Demux2/2 -> While Iterator Subsystem/2(Iteration)  "SCI_Tx_Iteration"
  Data_Logging/1(SCI_Tx) -> Demux2/1
  Data/1 -> Data_Conditioning_Tx/1(Data)

== system mcb_ipmsm_pos_est_f28379d/Embedded System/Initial Position Estimation (IPE) Algorithm/SCI_Tx/Simulation ==
  Data : Inport
  Terminator : Terminator
  wires:
  Data/1 -> Terminator/1

== system mcb_ipmsm_pos_est_f28379d/Embedded System/Initial Position Estimation (IPE) Algorithm/Scaling and Output/HW_Outputs ==
  Inverter Signals : Inport
  Code Generation : Subsystem  VariantControl=(codegen)
  Simulation : Subsystem  VariantControl=(sim)
  Sim : Outport

== system mcb_ipmsm_pos_est_f28379d/Embedded System/Initial Position Estimation (IPE) Algorithm/Scaling and Output/Output Scaling ==
  Vabc_ref : Inport
  Enable : Inport  Port=2
  Constant : Constant  Value=0.5  OutDataTypeStr=dataType  SampleTime=-1
  Data Type Conversion : DataTypeConversion  OutDataTypeStr=dataType  SaturateOnIntegerOverflow=off  RndMeth=Floor
  One_by_Two : Gain  Gain=0.5  RndMeth=Simplest  OutDataTypeStr=Inherit: Same as input
  Sum : Sum  Inputs=|++
  PWM_Duty_Cycles : Outport
  PWM_Enable : Outport  Port=2
  wires:
  Constant/1 -> Sum/2
  Sum/1 -> PWM_Duty_Cycles/1  "PWM_Duty_Cycles"
  One_by_Two/1 -> Sum/1
  Data Type Conversion/1 -> PWM_Enable/1
  Vabc_ref/1 -> One_by_Two/1
  Enable/1 -> Data Type Conversion/1

== system mcb_ipmsm_pos_est_f28379d/Embedded System/Serial Receive/Data_Conditioning_Rx/Data_Type_Fixed_Point ==
  In1 : Inport
  Data Type Conversion5 : DataTypeConversion  OutDataTypeStr=uint16  RndMeth=Simplest  SaturateOnIntegerOverflow=off
  Demux : Demux  Outputs=1
  Out3 : Outport
  wires:
  In1/1 -> Demux/1
  Data Type Conversion5/1 -> Out3/1
  Demux/1 -> Data Type Conversion5/1

== system mcb_ipmsm_pos_est_f28379d/Embedded System/Serial Receive/Data_Conditioning_Rx/Data_Type_Float ==
  In1 : Inport
  Data Type Conversion3 : DataTypeConversion  OutDataTypeStr=uint16  RndMeth=Simplest  SaturateOnIntegerOverflow=off
  Demux : Demux  Outputs=1
  Out3 : Outport
  wires:
  In1/1 -> Demux/1
  Data Type Conversion3/1 -> Out3/1
  Demux/1 -> Data Type Conversion3/1

== system mcb_ipmsm_pos_est_f28379d/Embedded System/Serial Receive/SCi_Rx/Code Generation ==
  Data_Type_Fixed_Point : Subsystem  VariantControl=~isequal(dataType, 'single')
  Data_Type_Float : Subsystem  VariantControl=isequal(dataType, 'single')
  Data : Outport

== system mcb_ipmsm_pos_est_f28379d/Embedded System/Serial Receive/SCi_Rx/Simulation ==
  Add1 : Sum  Commented=on  Inputs=+++
  Constant : Constant
  Data Type Conversion2 : DataTypeConversion  OutDataTypeStr=dataType  RndMeth=Simplest  SaturateOnIntegerOverflow=off
  Data_Conditioning_Tx1 : Subsystem  Variant=on
  Step2 : Step  Commented=on  Time=0.1
  Step3 : Step  Commented=on  Time=0.4  After=-1
  Step4 : Step  Commented=on  Time=0.5
  Data : Outport
  wires:
  Data_Conditioning_Tx1/1(Data) -> Data/1
  Data Type Conversion2/1 -> Data_Conditioning_Tx1/1(In1)
  Step2/1 -> Add1/1
  Step3/1 -> Add1/2
  Step4/1 -> Add1/3
  Constant/1 -> Data Type Conversion2/1

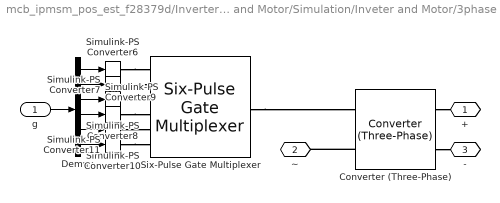
== system mcb_ipmsm_pos_est_f28379d/Inverter and Motor/Simulation/Inveter and Motor/3phase converter ==
  g : Inport
  Converter (Three-Phase) : ee_lib/Semiconductors & Converters/Converters/Converter (Three-Phase)  port_option=ee.enum.threePhasePort.composite  device_type=ee.enum.converters.switchingdevice.ideal  K=0  Vf=0.8 V  Ron=0.001 Ohm  Rds=0.001 Ohm  Goff=1e-6 1/Ohm  Vgt=1 V  Vgt_off=-1 V  Ih=1 A  Vth=0.5 V  diode_param=ee.enum.converters.protectiondiode.none  diode_Vf=0.8 V  diode_Ron=0.001 Ohm  diode_Goff=1e-5 1/Ohm  diode_C=50 nF  diode_iRM=-235 A  diode_iF=300 A  diode_idot=-50 A/us  diode_trr_param=ee.enum.converters.diodetrr.trr_factor  diode_trr_factor=3  diode_trr=15 us  diode_Qrr=1500 s*uA  snubber_type=ee.enum.converters.snubber.exclude  Cs=1e-7 F  Rs=0.1 Ohm
  Demux : Demux  Outputs=6
  Simulink-PS Converter{6..11} (6 alike) : nesl_utility/Simulink-PS Converter  PhysicalDomain=network_engine_domain  SubClassName=ps_input  LeftPortType=input  RightPortType=output  PseudoPeriodic=off  Frequencies=[]  NoiseDistribution=none  NoiseParameters=[]  Unit=1  AffineConversion=off  FilteringAndDerivatives=provide  SimscapeFilterOrder=1  InputFilterTimeConstant=0.001  UdotUserProvided=0
  Six-Pulse Gate Multiplexer : ee_lib/Semiconductors & Converters/Converters/Six-Pulse Gate Multiplexer  port_option=ee.enum.controlport.ps
  + : PMIOPort  Side=Right
  ~ : PMIOPort  Port=2  Side=Left
  - : PMIOPort  Port=3  Side=Right
  wires:
  g/1 -> Demux/1
  Demux/1 -> Simulink-PS Converter6/1
  Demux/2 -> Simulink-PS Converter7/1
  Demux/3 -> Simulink-PS Converter8/1
  Demux/4 -> Simulink-PS Converter9/1
  Demux/6 -> Simulink-PS Converter11/1
  Demux/5 -> Simulink-PS Converter10/1
  connections:
  Simulink-PS Converter6/RConn1 -- Six-Pulse Gate Multiplexer/LConn1
  Converter (Three-Phase)/RConn2 -- -/RConn1
  Converter (Three-Phase)/RConn1 -- +/RConn1
  Converter (Three-Phase)/LConn2 -- ~/RConn1
  Six-Pulse Gate Multiplexer/RConn1 -- Converter (Three-Phase)/LConn1
  Simulink-PS Converter7/RConn1 -- Six-Pulse Gate Multiplexer/LConn2
  Simulink-PS Converter8/RConn1 -- Six-Pulse Gate Multiplexer/LConn3
  Simulink-PS Converter9/RConn1 -- Six-Pulse Gate Multiplexer/LConn4
  Simulink-PS Converter10/RConn1 -- Six-Pulse Gate Multiplexer/LConn5
  Simulink-PS Converter11/RConn1 -- Six-Pulse Gate Multiplexer/LConn6

== system mcb_ipmsm_pos_est_f28379d/Inverter and Motor/Simulation/Inveter and Motor/6-pulse PWM generator ==
  ModWave : Inport
  Data Type Conversion : DataTypeConversion  SaturateOnIntegerOverflow=off  RndMeth=Floor
  Mux : Mux  Inputs=2
  NOT : Logic  Operator=NOT  IconShape=distinctive  AllPortsSameDT=off  OutDataTypeStr=boolean
  Relay : Relay
  Repeating Sequence Interpolated : simulink/Sources/Repeating Sequence Interpolated  OutValues=[0 1 0 -1 0].'  TimeValues=0.25/fs*[0 1 2 3 4].'  LookUpMeth=Interpolation-Use End Values  tsamp=Ts_motor_simscape  OutMin=[]  OutMax=[]  OutDataTypeStr=double  OutputDataTypeScalingMode=double  OutDataType=fixdt(0,8)  OutScaling=2^-10
  Selector : Selector  InputPortWidth=6  IndexOptions=Index vector (dialog)  Indices=[1 4 2 5 3 6]  OutputSizes=1
  Sum : Sum  Inputs=|+-
  g : Outport
  wires:
  Selector/1 -> g/1
  Mux/1 -> Selector/1
  Repeating Sequence Interpolated/1 -> Sum/2  "carrier"
  Sum/1 -> Relay/1
  Relay/1 -> Mux/1, NOT/1
  NOT/1 -> Data Type Conversion/1
  ModWave/1 -> Sum/1
  Data Type Conversion/1 -> Mux/2

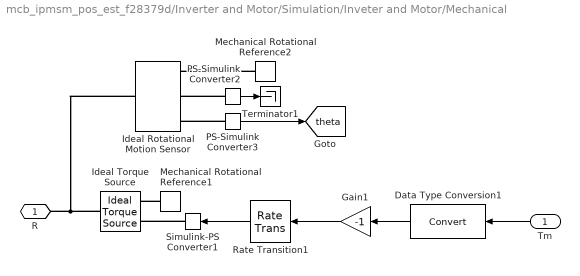
== system mcb_ipmsm_pos_est_f28379d/Inverter and Motor/Simulation/Inveter and Motor/Mechanical ==
  Tm : Inport
  Data Type Conversion1 : DataTypeConversion  SaturateOnIntegerOverflow=off  RndMeth=Floor
  Gain1 : Gain  Gain=-1
  Ideal Rotational Motion Sensor : fl_lib/Mechanical/Mechanical Sensors/Ideal Rotational Motion Sensor  reference=foundation.enum.MeasurementReference.difference  acceleration_port=false  velocity_port=true  position_port=true  wrap_angle=simscape.enum.onoff.on  offset=init_ang rad
  Ideal Torque Source : fl_lib/Mechanical/Mechanical Sources/Ideal Torque Source
  Mechanical Rotational Reference1 : fl_lib/Mechanical/Rotational Elements/Mechanical Rotational Reference
  Mechanical Rotational Reference2 : fl_lib/Mechanical/Rotational Elements/Mechanical Rotational Reference
  PS-Simulink Converter2 : nesl_utility/PS-Simulink Converter  PhysicalDomain=network_engine_domain  SubClassName=ps_output  LeftPortType=input  RightPortType=output  PseudoPeriodic=off  Frequencies=[]  VectorFormat=1-D array  Unit=rpm  AffineConversion=off
  PS-Simulink Converter3 : nesl_utility/PS-Simulink Converter  PhysicalDomain=network_engine_domain  SubClassName=ps_output  LeftPortType=input  RightPortType=output  PseudoPeriodic=off  Frequencies=[]  VectorFormat=1-D array  Unit=inherit  AffineConversion=off
  Rate Transition1 : RateTransition
  Simulink-PS Converter1 : nesl_utility/Simulink-PS Converter  PhysicalDomain=network_engine_domain  SubClassName=ps_input  LeftPortType=input  RightPortType=output  PseudoPeriodic=off  Frequencies=[]  NoiseDistribution=none  NoiseParameters=[]  Unit=N*m  AffineConversion=off  FilteringAndDerivatives=provide  SimscapeFilterOrder=1  InputFilterTimeConstant=0.001  UdotUserProvided=0
  Terminator1 : Terminator
  "R " : PMIOPort  Side=Right
  tag scope: theta=global
  wires:
  Gain1/1 -> Rate Transition1/1
  Data Type Conversion1/1 -> Gain1/1
  Tm/1 -> Data Type Conversion1/1
  PS-Simulink Converter2/1 -> Terminator1/1
  PS-Simulink Converter3/1 -> [theta]
  Rate Transition1/1 -> Simulink-PS Converter1/1
  connections:
  Mechanical Rotational Reference1/LConn1 -- Ideal Torque Source/RConn2
  Simulink-PS Converter1/RConn1 -- Ideal Torque Source/RConn1
  Ideal Torque Source/LConn1 -- Ideal Rotational Motion Sensor/LConn1 -- "R "/RConn1
  PS-Simulink Converter2/LConn1 -- Ideal Rotational Motion Sensor/RConn2
  PS-Simulink Converter3/LConn1 -- Ideal Rotational Motion Sensor/RConn3
  Mechanical Rotational Reference2/LConn1 -- Ideal Rotational Motion Sensor/RConn1

== system mcb_ipmsm_pos_est_f28379d/Inverter and Motor/Simulation/Inveter and Motor/Scale ==
  duty_abc : Inport
  Constant : Constant  Value=-0.5  OutDataTypeStr=double  SampleTime=Ts_motor_simscape
  Gain : Gain  Gain=2
  Rate Transition : RateTransition
  Sum : Sum  Inputs=|++
  ModWave : Outport
  wires:
  Sum/1 -> Gain/1
  Constant/1 -> Sum/2
  Rate Transition/1 -> ModWave/1  "ModWave"
  duty_abc/1 -> Sum/1
  Gain/1 -> Rate Transition/1

== system mcb_ipmsm_pos_est_f28379d/Inverter and Motor/Simulation/Inveter and Motor/measVI ==
  Current Sensor (Three-Phase) : ee_lib/Sensors & Transducers/Current Sensor (Three-Phase)
  Gain : Gain  Gain=pmsm.CurrFactor
  Line Voltage Sensor (Three-Phase) : ee_lib/Sensors & Transducers/Line Voltage Sensor (Three-Phase)
  PS-Simulink Converter4 : nesl_utility/PS-Simulink Converter  PhysicalDomain=network_engine_domain  SubClassName=ps_output  LeftPortType=input  RightPortType=output  PseudoPeriodic=off  Frequencies=[]  VectorFormat=1-D array  Unit=inherit  AffineConversion=off
  PS-Simulink Converter5 : nesl_utility/PS-Simulink Converter  PhysicalDomain=network_engine_domain  SubClassName=ps_output  LeftPortType=input  RightPortType=output  PseudoPeriodic=off  Frequencies=[]  VectorFormat=1-D array  Unit=inherit  AffineConversion=off
  ~1 : PMIOPort  Side=Left
  ~2 : PMIOPort  Port=2  Side=Right
  tag scope: Iabc=global, Vabc=global
  wires:
  PS-Simulink Converter5/1 -> [Vabc]  "Vabc"
  PS-Simulink Converter4/1 -> Gain/1  "Iabc"
  Gain/1 -> [Iabc]
  connections:
  PS-Simulink Converter4/LConn1 -- Current Sensor (Three-Phase)/RConn1
  PS-Simulink Converter5/LConn1 -- Line Voltage Sensor (Three-Phase)/RConn1
  Current Sensor (Three-Phase)/RConn2 -- ~2/RConn1
  Line Voltage Sensor (Three-Phase)/LConn1 -- ~1/RConn1 -- Current Sensor (Three-Phase)/LConn1

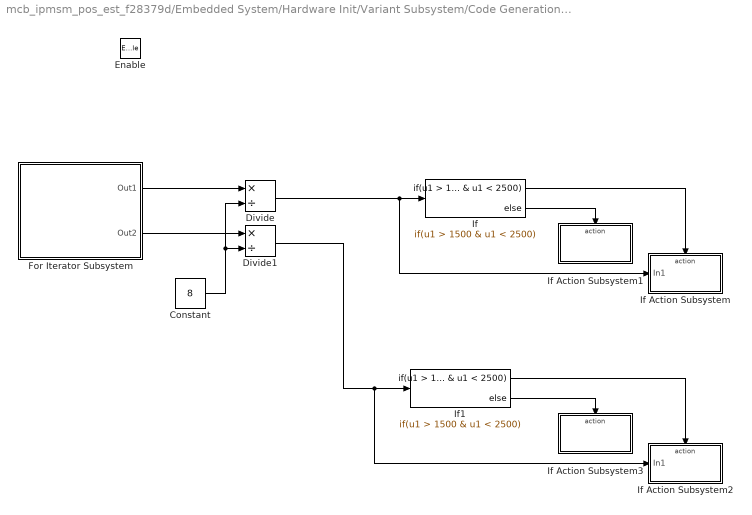
== system mcb_ipmsm_pos_est_f28379d/Embedded System/Hardware Init/Variant Subsystem/Code Generation/Calculate ADC Offset  ==
  Enable : EnablePort
  Constant : Constant  Value=8
  Divide : Product  Inputs=*/  OutDataTypeStr=uint16
  Divide1 : Product  Inputs=*/  OutDataTypeStr=uint16
  For Iterator Subsystem : Subsystem  TreatAsAtomicUnit=on
  If : If  IfExpression=u1 > 1500 & u1 < 2500
  If Action Subsystem : Subsystem  TreatAsAtomicUnit=on
  If Action Subsystem1 : Subsystem  TreatAsAtomicUnit=on
  If Action Subsystem2 : Subsystem  TreatAsAtomicUnit=on
  If Action Subsystem3 : Subsystem  TreatAsAtomicUnit=on
  If1 : If  IfExpression=u1 > 1500 & u1 < 2500
  wires:
  For Iterator Subsystem/2(Out2) -> Divide1/1
  Divide/1 -> If Action Subsystem/1(In1), If/1
  For Iterator Subsystem/1(Out1) -> Divide/1
  Constant/1 -> Divide/2, Divide1/2
  Divide1/1 -> If Action Subsystem2/1(In1), If1/1
  If/1 -> If Action Subsystem/Action
  If/2 -> If Action Subsystem1/Action
  If1/1 -> If Action Subsystem2/Action
  If1/2 -> If Action Subsystem3/Action

== system mcb_ipmsm_pos_est_f28379d/Embedded System/Hardware Init/Variant Subsystem/Code Generation/DRV Enable ==
  note: Enable inverter
  In : Inport
  ADC Gain setting : Subsystem
  Constant : Constant  Value=inverter.EnableLogic
  Digital Output : c2837xDlib/Digital Output  Priority=10  GPIO_Number=GPIO120~GPIO127  GPIO_Bit0=off  GPIO_BIT0_Toggle=off  GPIO_Bit1=off  GPIO_BIT1_Toggle=off  GPIO_Bit2=off  GPIO_BIT2_Toggle=off  GPIO_Bit3=off  GPIO_BIT3_Toggle=off  GPIO_Bit4=on  GPIO_BIT4_Toggle=off  GPIO_Bit5=off  GPIO_BIT5_Toggle=off  GPIO_Bit6=off  GPIO_BIT6_Toggle=off  GPIO_Bit7=off  GPIO_BIT7_Toggle=off
  Digital Output1 : c2837xDlib/Digital Output  Priority=10  GPIO_Number=GPIO16~GPIO23  GPIO_Bit0=off  GPIO_BIT0_Toggle=off  GPIO_Bit1=off  GPIO_BIT1_Toggle=off  GPIO_Bit2=off  GPIO_BIT2_Toggle=off  GPIO_Bit3=off  GPIO_BIT3_Toggle=off  GPIO_Bit4=off  GPIO_BIT4_Toggle=off  GPIO_Bit5=off  GPIO_BIT5_Toggle=off  GPIO_Bit6=on  GPIO_BIT6_Toggle=off  GPIO_Bit7=off  GPIO_BIT7_Toggle=off
  Inverter Enable : Constant  OutDataTypeStr=uint16  SampleTime=-1
  NOT : Logic  Operator=NOT  IconShape=distinctive  AllPortsSameDT=off  OutDataTypeStr=boolean
  RunTimeMeasurement : Constant  OutDataTypeStr=uint16  SampleTime=-1
  Switch : Switch  Criteria=u2 > Threshold  SaturateOnIntegerOverflow=off  InputSameDT=off
  wires:
  Inverter Enable/1 -> Switch/1, NOT/1  "Active high logic for inverter enable"
  RunTimeMeasurement/1 -> Digital Output1/1
  Constant/1 -> ADC Gain setting/Enable, Switch/2
  Switch/1 -> Digital Output/1
  NOT/1 -> Switch/3  "Active low logic for inverter enable"
  In/1 -> ADC Gain setting/1(In1)

== system mcb_ipmsm_pos_est_f28379d/Embedded System/Hardware Init/Variant Subsystem/Code Generation/Default ADC Offset ==
  Enable : EnablePort
  Constant : Constant  Value=inverter.CtSensAOffset  OutDataTypeStr=Inherit: Inherit via back propagation
  Constant1 : Constant  Value=inverter.CtSensBOffset  OutDataTypeStr=Inherit: Inherit via back propagation
  Data Store Write1 : DataStoreWrite  DataStoreName=IaOffset  IndexOptions=Index vector (dialog)  Indices=1  OutputSizes=1
  Data Store Write2 : DataStoreWrite  DataStoreName=IbOffset  IndexOptions=Index vector (dialog)  Indices=1  OutputSizes=1
  wires:
  Constant/1 -> Data Store Write1/1
  Constant1/1 -> Data Store Write2/1

== system mcb_ipmsm_pos_est_f28379d/Embedded System/Initial Position Estimation (IPE) Algorithm/Input and Scaling/HW_Inputs/Sensor Driver Blocks (codegen) ==
  Sim : Inport
  ADC_B_IN2 : c2802xlib/ADC  blkParamProc=C2000_Type4  ADCModule=B  samplingMode=Single sample mode  ADCResolution=12-bit (Single-ended input)  useSOC1=SOC0  useSOC2=SOC0_SOC1  SOCAcquisitionWindow=15  SOCTriggerSource=ePWM1_ADCSOCA  SOCInterruptTrigger=No ADCINT  Ts=-1  dType=uint16  postInterrupt=on  interruptSel=ADCINT1  ADCINTContinuous=on  endma=off  chdma=1  conv1=ADCINA0  conv2=ADCINA0 and ADCINB0  conv1_Type4=ADCIN2  conv2_Type4=ADCIN0 and ADCIN1
  ADC_C_IN2 : c2802xlib/ADC  blkParamProc=C2000_Type4  ADCModule=C  samplingMode=Single sample mode  ADCResolution=12-bit (Single-ended input)  useSOC1=SOC0  useSOC2=SOC0_SOC1  SOCAcquisitionWindow=15  SOCTriggerSource=ePWM1_ADCSOCA  SOCInterruptTrigger=No ADCINT  Ts=-1  dType=uint16  postInterrupt=on  interruptSel=ADCINT1  ADCINTContinuous=on  endma=off  chdma=1  conv1=ADCINA0  conv2=ADCINA0 and ADCINB0  conv1_Type4=ADCIN2  conv2_Type4=ADCIN0 and ADCIN1
  Mux1 : Mux  Inputs=2
  Terminator : Terminator
  Out : Outport
  wires:
  ADC_C_IN2/1 -> Mux1/1
  Mux1/1 -> Out/1
  ADC_B_IN2/1 -> Mux1/2
  Sim/1 -> Terminator/1

== system mcb_ipmsm_pos_est_f28379d/Embedded System/Initial Position Estimation (IPE) Algorithm/Input and Scaling/HW_Inputs/Sensor Driver Blocks (sim) ==
  Sim : Inport
  Out : Outport
  wires:
  Sim/1 -> Out/1

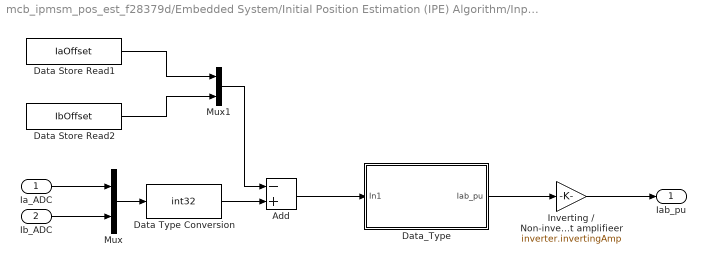
== system mcb_ipmsm_pos_est_f28379d/Embedded System/Initial Position Estimation (IPE) Algorithm/Input and Scaling/Input Scaling/Calculate Phase Currents ==
  Ia_ADC : Inport
  Ib_ADC : Inport  Port=2
  Add : Sum  Inputs=-+
  Data Store Read1 : DataStoreRead  DataStoreName=IaOffset  IndexOptions=Index vector (dialog)  Indices=1  OutputSizes=1
  Data Store Read2 : DataStoreRead  DataStoreName=IbOffset  IndexOptions=Index vector (dialog)  Indices=1  OutputSizes=1
  Data Type Conversion : DataTypeConversion  OutDataTypeStr=int32  ConvertRealWorld=Stored Integer (SI)  RndMeth=Simplest  SaturateOnIntegerOverflow=off
  Data_Type : Subsystem  Variant=on
  Inverting / Non-inverting Current measurement amplifieer : Gain  Gain=inverter.invertingAmp  RndMeth=Simplest  OutDataTypeStr=Inherit: Same as input
  Mux : Mux  Inputs=2
  Mux1 : Mux  Inputs=2
  Iab_pu : Outport  OutputWhenDisabled=reset  InitialOutput=[0 0]  VectorParamsAs1DForOutWhenUnconnected=off
  wires:
  Data Type Conversion/1 -> Add/2
  Data_Type/1(Iab_pu) -> Inverting / Non-inverting Current measurement amplifieer/1
  Ia_ADC/1 -> Mux/1
  Ib_ADC/1 -> Mux/2
  Mux/1 -> Data Type Conversion/1
  Data Store Read1/1 -> Mux1/1
  Data Store Read2/1 -> Mux1/2
  Mux1/1 -> Add/1
  Add/1 -> Data_Type/1(In1)
  Inverting / Non-inverting Current measurement amplifieer/1 -> Iab_pu/1

== system mcb_ipmsm_pos_est_f28379d/Embedded System/Initial Position Estimation (IPE) Algorithm/SCI_Tx/Code Generation/Data_Conditioning_Tx ==
  Data : Inport
  Data_Type_Fixed_Point : Subsystem  VariantControl=~isequal(dataType,'single')
  Data_Type_Float : Subsystem  VariantControl=isequal(dataType, 'single')
  Data_Log : Outport

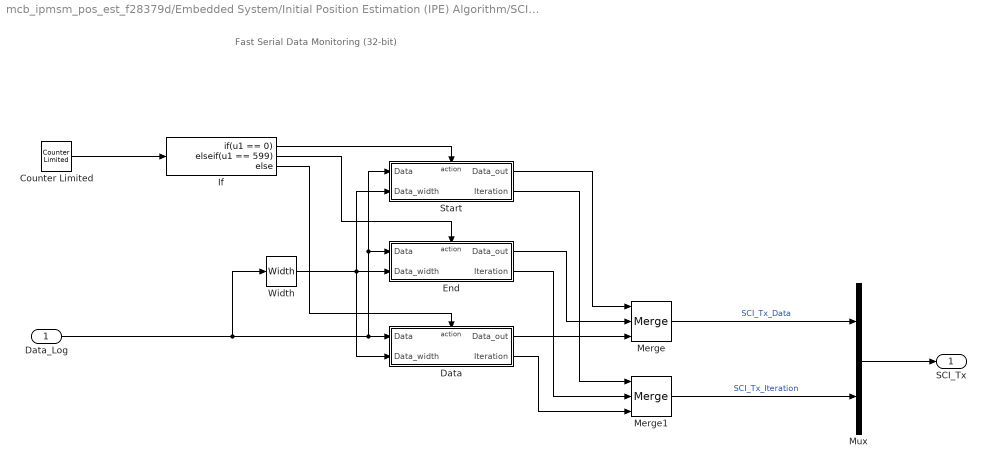
== system mcb_ipmsm_pos_est_f28379d/Embedded System/Initial Position Estimation (IPE) Algorithm/SCI_Tx/Code Generation/Data_Logging ==
  note: Fast Serial Data Monitoring (32-bit)
  Data_Log : Inport
  Counter Limited : simulink/Sources/Counter Limited  uplimit=600-1  tsamp=-1
  Data : Subsystem  TreatAsAtomicUnit=on
  End : Subsystem  TreatAsAtomicUnit=on
  If : If  IfExpression=u1 == 0  ElseIfExpressions=u1 == 599
  Merge : Merge  Inputs=3
  Merge1 : Merge  Inputs=3
  Mux : Mux  Inputs=2
  Start : Subsystem  TreatAsAtomicUnit=on
  Width : Width  OutDataTypeMode=All ports same datatype  DataType=uint16
  SCI_Tx : Outport
  wires:
  If/3 -> Data/Action
  Data/1(Data_out) -> Merge/3
  Width/1 -> Data/2(Data_width), Start/2(Data_width), End/2(Data_width)
  Merge/1 -> Mux/1  "SCI_Tx_Data"
  Counter Limited/1 -> If/1
  Start/2(Iteration) -> Merge1/1
  Start/1(Data_out) -> Merge/1
  If/2 -> End/Action
  Merge1/1 -> Mux/2  "SCI_Tx_Iteration"
  If/1 -> Start/Action
  End/1(Data_out) -> Merge/2
  End/2(Iteration) -> Merge1/2
  Data/2(Iteration) -> Merge1/3
  Mux/1 -> SCI_Tx/1
  Data_Log/1 -> Width/1, Start/1(Data), End/1(Data), Data/1(Data)

== system mcb_ipmsm_pos_est_f28379d/Embedded System/Initial Position Estimation (IPE) Algorithm/SCI_Tx/Code Generation/While Iterator Subsystem ==
  Data : Inport
  Iteration : Inport  Port=2
  Add : Sum  Inputs=+-  OutDataTypeStr=Inherit: Same as first input
  Index Vector : MultiPortSwitch  Inputs=1  SaturateOnIntegerOverflow=off  InputSameDT=off
  SCI Transmit : c280xlib/SCI Transmit  sciModule=A  dataHead=''  dataTail=''  frameSize=1  blockingMode=on  outputStatus=off
  While Iterator : WhileIterator  MaxIters=-1  WhileBlockType=do-while  ShowIterationPort=on  OutputDataType=int16
  wires:
  While Iterator/1 -> Add/2, Index Vector/1
  Data/1 -> Index Vector/2
  Index Vector/1 -> SCI Transmit/1
  Add/1 -> While Iterator/1
  Iteration/1 -> Add/1
